simulink model "bias_test"  (Simulink 9.0)
settings: Solver=FixedStepAuto  StartTime=0.0  StopTime=0  FixedStep=0.200000  MaxStep=1  RelTol=1e-3  EnableMultiTasking=on
settings Model: SuppressorTable=22 serialization::archive 11 0 6 0 0 0 0 0  Creator=arnaud  LastModifiedBy=hbourbou
settings DataIOCC: LimitDataPoints=on  SaveFormat=Structure
settings DebuggingCC: UnderspecifiedInitializationDetection=Simplified  MergeDetectMultiDrivingBlocksExec=error  SolverPrmCheckMsg=warning
settings GRTTargetCC: GeneratePreprocessorConditionals=Disable all
settings ConfigComp: CovSFcnEnable=off

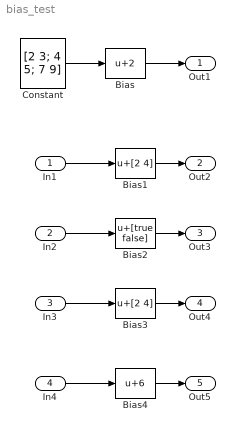
== system bias_test ==
  In1 : Inport
  In2 : Inport  Port=2
  In3 : Inport  Port=3  OutDataTypeStr=double
  In4 : Inport  Port=4  OutDataTypeStr=uint8  PortDimensions=3
  Bias : Bias  Bias=2
  Bias1 : Bias  Bias=[2 4]
  Bias2 : Bias  Bias=[true false]
  Bias3 : Bias  Bias=[2 4]
  Bias4 : Bias  Bias=6
  Constant : Constant  Value=[2 3; 4 5; 7 9]
  Out1 : Outport
  Out2 : Outport  Port=2
  Out3 : Outport  Port=3
  Out4 : Outport  Port=4
  Out5 : Outport  Port=5
  wires:
  Constant/1 -> Bias/1
  Bias/1 -> Out1/1
  In1/1 -> Bias1/1
  Bias1/1 -> Out2/1
  In2/1 -> Bias2/1
  Bias2/1 -> Out3/1
  In3/1 -> Bias3/1
  Bias3/1 -> Out4/1
  In4/1 -> Bias4/1
  Bias4/1 -> Out5/1
